simulink model "DifferenceRCequation"  (R2017a)
settings: Solver=VariableStepAuto  StartTime=0.0  StopTime=10.0  RelTol=1e-3
settings Model: Creator=Administrator  LastModifiedBy=Administrator

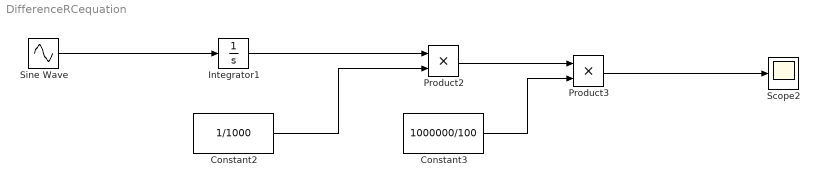
== system DifferenceRCequation ==
  Constant2 : Constant  Value=1/1000
  Constant3 : Constant  Value=1000000/100
  Integrator1 : Integrator
  Product2 : Product
  Product3 : Product
  Scope2 : Scope
  Sine Wave : Sin  SampleTime=0
  wires:
  Constant2/1 -> Product2/2
  Product3/1 -> Scope2/1
  Integrator1/1 -> Product2/1
  Constant3/1 -> Product3/2
  Product2/1 -> Product3/1
  Sine Wave/1 -> Integrator1/1
